simulink model "MondeoDP"  (Simulink 4.00)
settings: Solver=ode4  StartTime=t_0  StopTime=t_end  FixedStep=T_s  RelTol=1e-3
values from neighbouring files (symbols this model uses):
  a = 0.00005    (= 5e-05)    [MondeoBattData.m]
  GangZahl = Gang(k-1)    [dp.m]    (also in dp1.m; dp2.m)
  LadungAnfang = InitialCharge    [DP3.m]    (also in DP4.m = 0; DP5.m; DPVorwaerts.m; DPVorwaerts1.m)
  Mb = [0 0 0 0 0 0 0 0 0 0 0 0 ... (200 elements, 1x200)]    [MondemoECETraj.mat]    (also in MondemoTraj.mat = [0 0 0 0 0 0 0 0 0 0 0 0 ... (1181 elements, 1x1181)]; NeueTraj.m = [Mb V]; dp.m = MbOpt; dp1.m = MbOpt)
  Mv = Mp(k)    [DP3.m]    (also in DP4.m; DP5.m; DPVorwaerts.m; DPVorwaerts1.m)
  P_Load = 1000    [dp.m]    (also in dp1.m; dp2.m)
  Pe = 0    [DP3.m]    (also in dp1.m = PeOpt; dp2.m = PeOpt)
  SlipStick = 0    [dp1.m]    (also in dp2.m)
undefined symbols (not defined in the file or in its folder): B_Kap, B_Sp, magnitude
libraries: lib_driveline_components x10, lib_VES_components x2, simulink3 x1
settings Model: LastModifiedBy=meifert  BlockReductionOpt=off

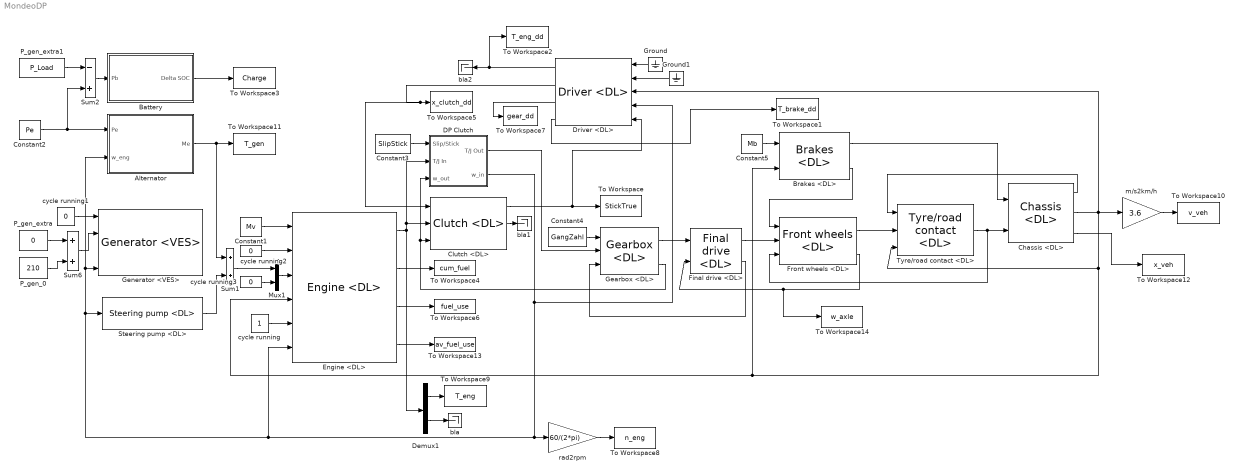
== system MondeoDP ==
  Alternator : Subsystem
      settings: RTWFcnNameOpts=Auto  RTWFileNameOpts=Auto
  Battery : Subsystem
      settings: RTWFcnNameOpts=Auto  RTWFileNameOpts=Auto
  Brakes <DL> : lib_driveline_components/Brakes <DL>  AncestorBlock=|
      | lib_wheel/wheel and
      | axle <wh>/front/rear brake controller interface
      | (achievable)
      settings: RTWFcnNameOpts=Auto  RTWFileNameOpts=Auto
  Chassis <DL> : lib_driveline_components/Chassis <DL>
      settings: RTWFcnNameOpts=Auto  RTWFileNameOpts=Auto
  Clutch <DL> : lib_driveline_components/Clutch <DL>
      settings: RTWFcnNameOpts=Auto  RTWFileNameOpts=Auto
  Constant1 : Constant  Value=Mv
  Constant2 : Constant  Value=Pe
  Constant3 : Constant  Value=SlipStick
  Constant4 : Constant  Value=GangZahl
  Constant5 : Constant  Value=Mb
  DP Clutch : Subsystem
      settings: RTWFcnNameOpts=Auto  RTWFileNameOpts=Auto
  Demux1 : Demux  Outputs=2  BusSelectionMode=off
  Driver <DL> : lib_driveline_components/Driver <DL>  Orientation=left
      settings: RTWFcnNameOpts=Auto  RTWFileNameOpts=Auto
  Engine <DL> : lib_driveline_components/Engine <DL>
      settings: RTWFcnNameOpts=Auto  RTWFileNameOpts=Auto
  Final drive <DL> : lib_driveline_components/Final drive <DL>
      settings: RTWFcnNameOpts=Auto  RTWFileNameOpts=Auto
  Front wheels <DL> : lib_driveline_components/Front wheels <DL>
      settings: RTWFcnNameOpts=Auto  RTWFileNameOpts=Auto
  Gearbox <DL> : lib_driveline_components/Gearbox <DL>
      settings: RTWFcnNameOpts=Auto  RTWFileNameOpts=Auto
  Generator <VES> : lib_VES_components/Generator <VES>
      settings: RTWFcnNameOpts=Auto  RTWFileNameOpts=Auto
  Ground : Ground  Orientation=left
  Ground1 : Ground  Orientation=left
  Mux1 : Mux  Inputs=2
  P_gen_0 : Constant  Value=210
  P_gen_extra : Constant  Value=0
  P_gen_extra1 : Constant  Value=P_Load
  Steering pump <DL> : lib_driveline_components/Steering pump <DL>
      settings: RTWFcnNameOpts=Auto  RTWFileNameOpts=Auto
  Sum1 : Sum  Inputs=++  SaturateOnIntegerOverflow=on
  Sum2 : Sum  Inputs=-+  SaturateOnIntegerOverflow=on
  Sum6 : Sum  Inputs=++  SaturateOnIntegerOverflow=on
  To Workspace : ToWorkspace  VariableName=StickTrue  SampleTime=-1  SaveFormat=Array
  To Workspace1 : ToWorkspace  VariableName=T_brake_dd  SampleTime=-1  SaveFormat=Array
  To Workspace10 : ToWorkspace  VariableName=v_veh  SampleTime=-1  SaveFormat=Array
  To Workspace11 : ToWorkspace  VariableName=T_gen  SampleTime=-1  SaveFormat=Array
  To Workspace12 : ToWorkspace  VariableName=x_veh  SampleTime=-1  SaveFormat=Array
  To Workspace13 : ToWorkspace  VariableName=av_fuel_use  SampleTime=-1  SaveFormat=Array
  To Workspace14 : ToWorkspace  VariableName=w_axle  SampleTime=-1  SaveFormat=Array
  To Workspace2 : ToWorkspace  VariableName=T_eng_dd  SampleTime=-1  SaveFormat=Array
  To Workspace3 : ToWorkspace  VariableName=Charge  SampleTime=-1  SaveFormat=Array
  To Workspace4 : ToWorkspace  VariableName=cum_fuel  SampleTime=-1  SaveFormat=Array
  To Workspace5 : ToWorkspace  VariableName=x_clutch_dd  SampleTime=-1  SaveFormat=Array
  To Workspace6 : ToWorkspace  VariableName=fuel_use  SampleTime=-1  SaveFormat=Array
  To Workspace7 : ToWorkspace  VariableName=gear_dd  SampleTime=-1  SaveFormat=Array
  To Workspace8 : ToWorkspace  VariableName=n_eng  SampleTime=-1  SaveFormat=Array
  To Workspace9 : ToWorkspace  VariableName=T_eng  SampleTime=-1  SaveFormat=Array
  Tyre/road contact <DL> : lib_driveline_components/Tyre//road contact <DL>
      settings: RTWFcnNameOpts=Auto  RTWFileNameOpts=Auto
  bla : Terminator
  bla1 : Terminator
  bla2 : Terminator
  cycle running : Constant  Value=1
  cycle running1 : Constant  Value=0
  cycle running2 : Constant  Value=0
  cycle running3 : Constant  Value=0
  m/s2km/h : Gain  Gain=3.6  Multiplication=Element-wise(K.*u)  SaturateOnIntegerOverflow=on
  rad2rpm : Gain  Gain=60/(2*pi)  Multiplication=Element-wise(K.*u)  SaturateOnIntegerOverflow=on
  wires:
  Gearbox <DL>/1 -> Final drive <DL>/1
  Final drive <DL>/2 -> Gearbox <DL>/3
  Chassis <DL>/2 -> Driver <DL>/3, Tyre/road contact <DL>/3, Brakes <DL>/2, Engine <DL>/4, m/s2km/h/1
  Front wheels <DL>/2 -> Final drive <DL>/2, To Workspace14/1
  rad2rpm/1 -> To Workspace8/1
  Demux1/1 -> To Workspace9/1
  Demux1/2 -> bla/1
  Driver <DL>/1 -> To Workspace2/1, bla2/1
  Driver <DL>/2 -> To Workspace5/1, Clutch <DL>/1
  Driver <DL>/3 -> To Workspace7/1
  m/s2km/h/1 -> To Workspace10/1
  Brakes <DL>/1 -> Chassis <DL>/1
  Tyre/road contact <DL>/1 -> Front wheels <DL>/3, Chassis <DL>/2
  Front wheels <DL>/1 -> Tyre/road contact <DL>/2
  Chassis <DL>/1 -> Tyre/road contact <DL>/1
  Gearbox <DL>/2 -> DP Clutch/3(w_out), Clutch <DL>/3
  DP Clutch/2(w_in) -> Driver <DL>/4, rad2rpm/1, Engine <DL>/6, Steering pump <DL>/1, Generator <VES>/4, Alternator/2(w_eng)
  Clutch <DL>/1 -> To Workspace/1, Driver <DL>/5
  Brakes <DL>/2 -> Front wheels <DL>/1
  Final drive <DL>/1 -> Front wheels <DL>/2
  Mux1/1 -> Engine <DL>/3
  Engine <DL>/1 -> Demux1/1, DP Clutch/2(T/J In), Clutch <DL>/2
  P_gen_extra/1 -> Sum6/1
  Engine <DL>/3 -> To Workspace6/1
  cycle running/1 -> Engine <DL>/5
  Engine <DL>/2 -> To Workspace4/1
  Chassis <DL>/3 -> To Workspace12/1
  Engine <DL>/4 -> To Workspace13/1
  P_gen_0/1 -> Sum6/2
  Sum1/1 -> Mux1/1
  Steering pump <DL>/1 -> Sum1/2
  cycle running1/1 -> Generator <VES>/1
  Sum6/1 -> Generator <VES>/2
  Constant3/1 -> DP Clutch/1(Slip/Stick)
  DP Clutch/1(T/J Out) -> Gearbox <DL>/2
  Clutch <DL>/2 -> bla1/1
  cycle running2/1 -> Engine <DL>/2
  cycle running3/1 -> Mux1/2
  Constant1/1 -> Engine <DL>/1
  Alternator/1(Me) -> Sum1/1, To Workspace11/1
  Constant2/1 -> Alternator/1(Pe), Sum2/2
  Constant4/1 -> Gearbox <DL>/1
  Driver <DL>/4 -> To Workspace1/1
  Constant5/1 -> Brakes <DL>/1
  Ground1/1 -> Driver <DL>/2
  Ground/1 -> Driver <DL>/1
  Sum2/1 -> Battery/1(Pb)
  P_gen_extra1/1 -> Sum2/1
  Battery/1(Delta SOC) -> To Workspace3/1

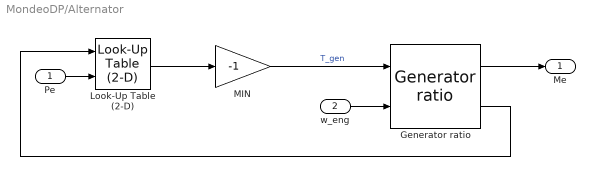
== system MondeoDP/Alternator ==
  Pe : Inport  Port=1  LatchInput=off
  w_eng : Inport  Port=2  LatchInput=off
  Generator ratio : lib_VES_components/Generator <VES>/Generator ratio
      settings: RTWFcnNameOpts=Auto  RTWFileNameOpts=Auto
  Look-Up Table (2-D) : simulink3/Functions & Tables/Look-Up Table (2-D)  x=gen_effmap_speeds  y=gen_effmap_Pels  t=gen_effmap_table
  MIN : Gain  Gain=-1  Multiplication=Element-wise(K.*u)  SaturateOnIntegerOverflow=on
  Me : Outport  Port=1
  wires:
  w_eng/1 -> Generator ratio/2
  Generator ratio/2 -> Look-Up Table (2-D)/1
  MIN/1 -> Generator ratio/1  "T_gen"
  Look-Up Table (2-D)/1 -> MIN/1
  Generator ratio/1 -> Me/1
  Pe/1 -> Look-Up Table (2-D)/2

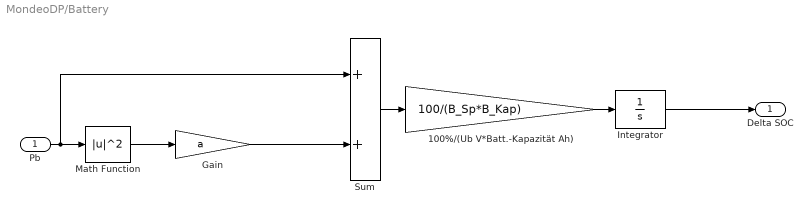
== system MondeoDP/Battery ==
  Pb : Inport  Port=1  LatchInput=off
  100%/(Ub V*Batt.-Kapazität Ah) : Gain  Gain=100/(B_Sp*B_Kap)  Multiplication=Element-wise(K.*u)  SaturateOnIntegerOverflow=on
  Gain : Gain  Gain=a  Multiplication=Element-wise(K.*u)  SaturateOnIntegerOverflow=on
  Integrator : Integrator  ExternalReset=none  InitialConditionSource=internal  InitialCondition=LadungAnfang  LimitOutput=off  UpperSaturationLimit=inf  LowerSaturationLimit=-inf  ShowSaturationPort=off  ShowStatePort=off  AbsoluteTolerance=auto
  Math Function : Math  Operator=magnitude^2  OutputSignalType=auto
  Sum : Sum  Inputs=++  SaturateOnIntegerOverflow=on
  Delta SOC : Outport  Port=1
  wires:
  Gain/1 -> Sum/2
  Math Function/1 -> Gain/1
  Pb/1 -> Math Function/1, Sum/1
  Sum/1 -> 100%/(Ub V*Batt.-Kapazität Ah)/1
  Integrator/1 -> Delta SOC/1
  100%/(Ub V*Batt.-Kapazität Ah)/1 -> Integrator/1

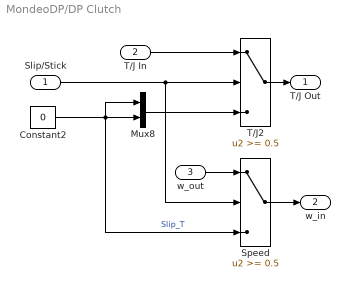
== system MondeoDP/DP Clutch ==
  Slip/Stick : Inport  Port=1  LatchInput=off
  T/J In : Inport  Port=2  LatchInput=off
  w_out : Inport  Port=3  LatchInput=off
  Constant2 : Constant  Value=0
  Mux8 : Mux  Inputs=2
      settings: DisplayOption=none
  Speed : Switch  Threshold=0.5
  T/J2 : Switch  Threshold=0.5
  T/J Out : Outport  Port=1
  w_in : Outport  Port=2
  wires:
  Constant2/1 -> Mux8/2, Mux8/1, Speed/3  "Slip_T"
  Mux8/1 -> T/J2/3
  T/J In/1 -> T/J2/1
  T/J2/1 -> T/J Out/1
  Slip/Stick/1 -> T/J2/2, Speed/2
  Speed/1 -> w_in/1
  w_out/1 -> Speed/1
